simulink model "NPPF_N2_TH4"  (Simulink 10.0)
settings: Solver=VariableStepAuto  StartTime=0.0  StopTime=50  RelTol=1e-3
undefined symbols (not defined in the file): AL1, AL2, AT1, AT2, b, d, disturbance, g, Ix, Iy, Iz, l, m, P1, P2, t_end, t_start
libraries: truetime x3, simulink x3
settings Model: Creator=sunny  LastModifiedBy=peter
settings DataIOCC: LimitDataPoints=on  SignalLoggingSaveFormat=ModelDataLogs
settings OptimizationCC: BlockReduction=off  BooleanDataType=off
settings DebuggingCC: SaveWithParameterizedLinksMsg=none  SignalResolutionControl=TryResolveAllWithWarning  MultiTaskDSMMsg=warning  MultiTaskCondExecSysMsg=none  StateNameClashWarn=warning
settings HardwareCC: TargetBitPerPointer=64  TargetBitPerSizeT=64  TargetBitPerPtrDiffT=64  TargetLongLongMode=on  TargetIntDivRoundTo=Zero  TargetEndianess=LittleEndian  TargetWordSize=64  TargetHWDeviceType=MATLAB Host  ProdEqTarget=off
settings GRTTargetCC: CombineOutputUpdateFcns=on  GRTInterface=off
settings ConfigComp: CovExternalEMLEnable=off

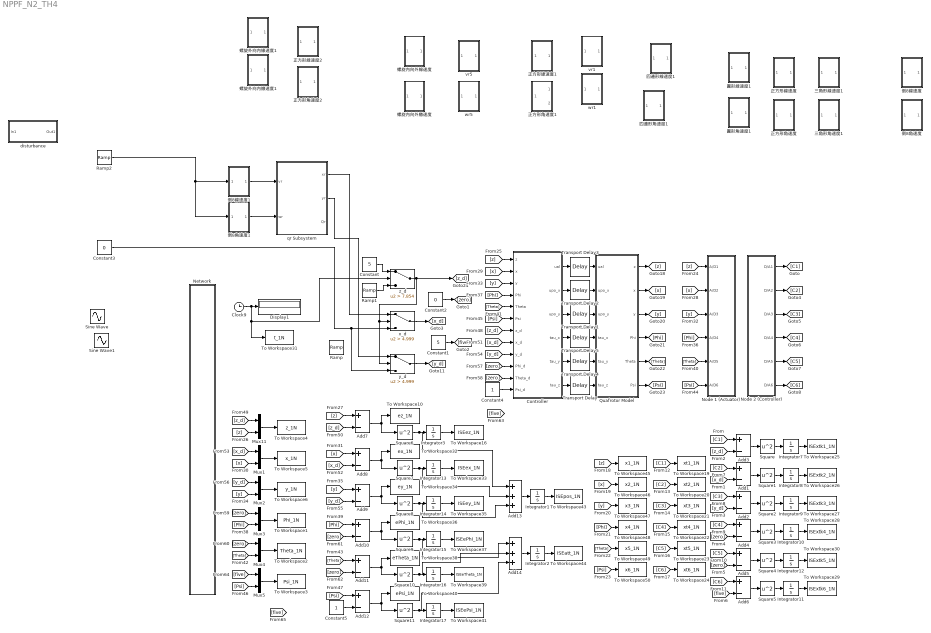
== system NPPF_N2_TH4 ==
  Add{1..12} (12 alike) : Sum  Inputs=+-
  Add13 : Sum  Inputs=+++
  Add14 : Sum  Inputs=+++
  Clock9 : Clock
  Constant : Constant  Value=5
  Constant1 : Constant  Value=5
  Constant2 : Constant  Value=0
  Constant3 : Constant  Value=0
  Constant4 : Constant
  Constant5 : Constant
  Controller : Subsystem
  Display1 : Display
  Integrator{1..3,7..17} (14 alike) : Integrator
  Mux{1..5,11} (6 alike) : Mux  Inputs=2
  Network : Subsystem
  Node 1 (Actuator) : Subsystem
  Node 2 (Controller) : Subsystem
  Quafrotor Model : Subsystem
  Ramp : simulink/Sources/Ramp  slope=0.5858/7.854  start=0  InitialOutput=0
  Ramp1 : simulink/Sources/Ramp  slope=5/7.854  start=0  InitialOutput=0
  Ramp2 : simulink/Sources/Ramp  slope=1  start=0  InitialOutput=0
  Sine Wave : Sin  Amplitude=2  Bias=2  Frequency=0.5  Phase=pi/2  SampleTime=0
  Sine Wave1 : Sin  Amplitude=2  Bias=2  Frequency=0.5  SampleTime=0
  Square{,1..11} (12 alike) : Math  Operator=square  SaturateOnIntegerOverflow=on
  To Workspace1 : ToWorkspace  VariableName=Phi_1N  SampleTime=-1
  To Workspace10 : ToWorkspace  VariableName=ez_1N  SampleTime=-1
  To Workspace16 : ToWorkspace  VariableName=ISEez_1N  SampleTime=-1
  To Workspace19 : ToWorkspace  VariableName=xt1_1N  SampleTime=-1
  To Workspace2 : ToWorkspace  VariableName=Theta_1N  SampleTime=-1
  To Workspace20 : ToWorkspace  VariableName=xt2_1N  SampleTime=-1
  To Workspace21 : ToWorkspace  VariableName=xt3_1N  SampleTime=-1
  To Workspace22 : ToWorkspace  VariableName=xt4_1N  SampleTime=-1
  To Workspace23 : ToWorkspace  VariableName=xt5_1N  SampleTime=-1
  To Workspace24 : ToWorkspace  VariableName=xt6_1N  SampleTime=-1
  To Workspace25 : ToWorkspace  VariableName=ISExtk1_1N  SampleTime=-1
  To Workspace26 : ToWorkspace  VariableName=ISExtk2_1N  SampleTime=-1
  To Workspace27 : ToWorkspace  VariableName=ISExtk3_1N  SampleTime=-1
  To Workspace28 : ToWorkspace  VariableName=ISExtk4_1N  SampleTime=-1
  To Workspace29 : ToWorkspace  VariableName=ISExtk6_1N  SampleTime=-1
  To Workspace3 : ToWorkspace  VariableName=Psi_1N  SampleTime=-1
  To Workspace30 : ToWorkspace  VariableName=ISExtk5_1N  SampleTime=-1
  To Workspace31 : ToWorkspace  VariableName=t_1N  SampleTime=-1
  To Workspace32 : ToWorkspace  VariableName=ex_1N  SampleTime=-1
  To Workspace33 : ToWorkspace  VariableName=ISEex_1N  SampleTime=-1
  To Workspace34 : ToWorkspace  VariableName=ey_1N  SampleTime=-1
  To Workspace35 : ToWorkspace  VariableName=ISEey_1N  SampleTime=-1
  To Workspace36 : ToWorkspace  VariableName=ePhi_1N  SampleTime=-1
  To Workspace37 : ToWorkspace  VariableName=ISEePhi_1N  SampleTime=-1
  To Workspace38 : ToWorkspace  VariableName=eTheta_1N  SampleTime=-1
  To Workspace39 : ToWorkspace  VariableName=ISEeTheta_1N  SampleTime=-1
  To Workspace4 : ToWorkspace  VariableName=z_1N  SampleTime=-1
  To Workspace40 : ToWorkspace  VariableName=ePsi_1N  SampleTime=-1
  To Workspace41 : ToWorkspace  VariableName=ISEePsi_1N  SampleTime=-1
  To Workspace43 : ToWorkspace  VariableName=ISEpos_1N  SampleTime=-1
  To Workspace44 : ToWorkspace  VariableName=ISEatt_1N  SampleTime=-1
  To Workspace45 : ToWorkspace  VariableName=x1_1N  SampleTime=-1
  To Workspace46 : ToWorkspace  VariableName=x2_1N  SampleTime=-1
  To Workspace47 : ToWorkspace  VariableName=x3_1N  SampleTime=-1
  To Workspace48 : ToWorkspace  VariableName=x4_1N  SampleTime=-1
  To Workspace49 : ToWorkspace  VariableName=x5_1N  SampleTime=-1
  To Workspace5 : ToWorkspace  VariableName=x_1N  SampleTime=-1
  To Workspace50 : ToWorkspace  VariableName=x6_1N  SampleTime=-1
  To Workspace6 : ToWorkspace  VariableName=y_1N  SampleTime=-1
  Transport Delay{,1..5} (6 alike) : TransportDelay
  disturbance : Subsystem
  qr Subsystem : Subsystem
  vr1 : Subsystem
  vr5 : Subsystem
  wr1 : Subsystem
  wr5 : Subsystem
  x_d : Switch  Criteria=u2 > Threshold  Threshold=4.999
  y_d : Switch  Criteria=u2 > Threshold  Threshold=4.999
  z_d : Switch  Criteria=u2 > Threshold  Threshold=7.854
  三角形線速度1 : Subsystem
  三角形角速度1 : Subsystem
  倒8線速度 : Subsystem
  倒8線速度1 : Subsystem
  倒8角速度 : Subsystem
  倒8角速度1 : Subsystem
  四邊形線速度1 : Subsystem
  四邊形角速度1 : Subsystem
  圓形線速度1 : Subsystem
  圓形角速度1 : Subsystem
  正方形線速度 : Subsystem
  正方形線速度1 : Subsystem
  正方形線速度2 : Subsystem
  正方形角速度 : Subsystem
  正方形角速度1 : Subsystem
  正方形角速度2 : Subsystem
  螺旋內向外線速度 : Subsystem
  螺旋內向外繳速度 : Subsystem
  螺旋外向內線速度1 : Subsystem
  螺旋外向內繳速度1 : Subsystem
  wires:
  Ramp1/1 -> z_d/3
  Constant/1 -> z_d/1
  Clock9/1 -> To Workspace31/1, z_d/2, Display1/1
  Controller/1(ual) -> Transport Delay3/1
  Controller/6(tau_z) -> Transport Delay/1
  Controller/5(tau_y) -> Transport Delay4/1
  Controller/4(tau_x) -> Transport Delay5/1
  Controller/3(upo_y) -> Transport Delay1/1
  Controller/2(upo_x) -> Transport Delay2/1
  Mux11/1 -> To Workspace4/1
  Integrator7/1 -> To Workspace25/1
  Square/1 -> Integrator7/1
  Add3/1 -> Square/1
  Add1/1 -> Square1/1
  Square1/1 -> Integrator8/1
  Integrator8/1 -> To Workspace26/1
  Square2/1 -> Integrator9/1
  Integrator9/1 -> To Workspace27/1
  Add2/1 -> Square2/1
  Integrator10/1 -> To Workspace28/1
  Square3/1 -> Integrator10/1
  Add4/1 -> Square3/1
  Add5/1 -> Square4/1
  Square4/1 -> Integrator12/1
  Integrator12/1 -> To Workspace30/1
  Add6/1 -> Square5/1
  Integrator11/1 -> To Workspace29/1
  Square5/1 -> Integrator11/1
  Integrator3/1 -> To Workspace16/1
  Square6/1 -> Add13/1, Integrator3/1
  Add7/1 -> Square6/1, To Workspace10/1
  Square7/1 -> Add13/2, Integrator13/1
  Add8/1 -> Square7/1, To Workspace32/1
  Integrator13/1 -> To Workspace33/1
  Integrator14/1 -> To Workspace35/1
  Square8/1 -> Add13/3, Integrator14/1
  Add9/1 -> Square8/1, To Workspace34/1
  Integrator15/1 -> To Workspace37/1
  Square9/1 -> Add14/1, Integrator15/1
  Add10/1 -> Square9/1, To Workspace36/1
  Integrator16/1 -> To Workspace39/1
  Square10/1 -> Add14/2, Integrator16/1
  Add11/1 -> Square10/1, To Workspace38/1
  Integrator17/1 -> To Workspace41/1
  Square11/1 -> Add14/3, Integrator17/1
  Add12/1 -> Square11/1, To Workspace40/1
  [z_d] -> Add3/2
  Node 2 (Controller)/1(D/A1) -> [C1]
  Node 2 (Controller)/2(D/A2) -> [C2]
  Node 2 (Controller)/3(D/A3) -> [C3]
  Node 2 (Controller)/4(D/A4) -> [C4]
  Node 2 (Controller)/5(D/A5) -> [C5]
  Node 2 (Controller)/6(D/A6) -> [C6]
  [C1] -> Add3/1
  [x_d] -> Add1/2
  [C2] -> Add1/1
  [C3] -> Add2/1
  [y_d] -> Add2/2
  [C4] -> Add4/1
  [zero] -> Add4/2
  [C5] -> Add5/1
  [zero] -> Add5/2
  [C6] -> Add6/1
  [five] -> Add6/2
  [C1] -> To Workspace19/1
  [C2] -> To Workspace20/1
  [C3] -> To Workspace21/1
  [C4] -> To Workspace22/1
  [C5] -> To Workspace23/1
  [C6] -> To Workspace24/1
  Quafrotor Model/1(z) -> [z]
  [z] -> Node 1 (Actuator)/1(A/D1)
  [z] -> Controller/1(z)
  [z] -> Mux11/2
  [z] -> Add7/1
  Quafrotor Model/2(x) -> [x]
  [x] -> Node 1 (Actuator)/2(A/D2)
  [x] -> Controller/2(x)
  [x] -> Add8/1
  Quafrotor Model/3(y) -> [y]
  [y] -> Node 1 (Actuator)/3(A/D3)
  [y] -> Controller/3(y)
  [y] -> Add9/1
  Quafrotor Model/4(Phi) -> [Phi]
  [Phi] -> Node 1 (Actuator)/4(A/D4)
  [Phi] -> Controller/4(Phi)
  [Phi] -> Add10/1
  Quafrotor Model/5(Theta) -> [Theta]
  [Theta] -> Node 1 (Actuator)/5(A/D5)
  [Theta] -> Controller/5(Theta)
  [Theta] -> Add11/1
  Quafrotor Model/6(Psi) -> [Psi]
  [Psi] -> Node 1 (Actuator)/6(A/D6)
  [Psi] -> Controller/6("Psi ")
  [Psi] -> Add12/1
  z_d/1 -> [z_d], y_d/2, x_d/2
  [z_d] -> Controller/7(z_d)
  [z_d] -> Mux11/1
  [z_d] -> Add7/2
  x_d/1 -> [x_d]
  [x_d] -> Controller/8(x_d)
  [x_d] -> Add8/2
  y_d/1 -> [y_d]
  [y_d] -> Controller/9(y_d)
  [y_d] -> Add9/2
  Constant2/1 -> [zero]
  Constant1/1 -> [five]
  [zero] -> Controller/10(Phi_d)
  [zero] -> Controller/11(Theta_d)
  [zero] -> Add10/2
  [zero] -> Add11/2
  Constant4/1 -> Controller/12(Psi_d)
  Constant5/1 -> Add12/2
  [x_d] -> Mux1/1
  Mux1/1 -> To Workspace5/1
  [x] -> Mux1/2
  [y_d] -> Mux2/1
  Mux2/1 -> To Workspace6/1
  [y] -> Mux2/2
  [zero] -> Mux3/1
  Mux3/1 -> To Workspace1/1
  [Phi] -> Mux3/2
  [zero] -> Mux4/1
  Mux4/1 -> To Workspace2/1
  [Theta] -> Mux4/2
  [five] -> Mux5/1
  Mux5/1 -> To Workspace3/1
  [Psi] -> Mux5/2
  Add13/1 -> Integrator1/1
  Integrator1/1 -> To Workspace43/1
  Add14/1 -> Integrator2/1
  Integrator2/1 -> To Workspace44/1
  [Psi] -> To Workspace50/1
  [z] -> To Workspace45/1
  [Phi] -> To Workspace48/1
  [y] -> To Workspace47/1
  [Theta] -> To Workspace49/1
  [x] -> To Workspace46/1
  倒8線速度1/1(Out1) -> qr Subsystem/1(vr)
  倒8角速度1/1(Out1) -> qr Subsystem/2(wr)
  Constant3/1 -> y_d/3, x_d/3
  qr Subsystem/1(xr) -> x_d/1
  qr Subsystem/2(yr) -> y_d/1
  Ramp2/1 -> 倒8角速度1/1(In2), 倒8線速度1/1(In2)
  Transport Delay3/1 -> Quafrotor Model/1(ual)
  Transport Delay2/1 -> Quafrotor Model/2(upo_x)
  Transport Delay1/1 -> Quafrotor Model/3(upo_y)
  Transport Delay5/1 -> Quafrotor Model/4(tau_x)
  Transport Delay4/1 -> Quafrotor Model/5(tau_y)
  Transport Delay/1 -> Quafrotor Model/6(tau_z)

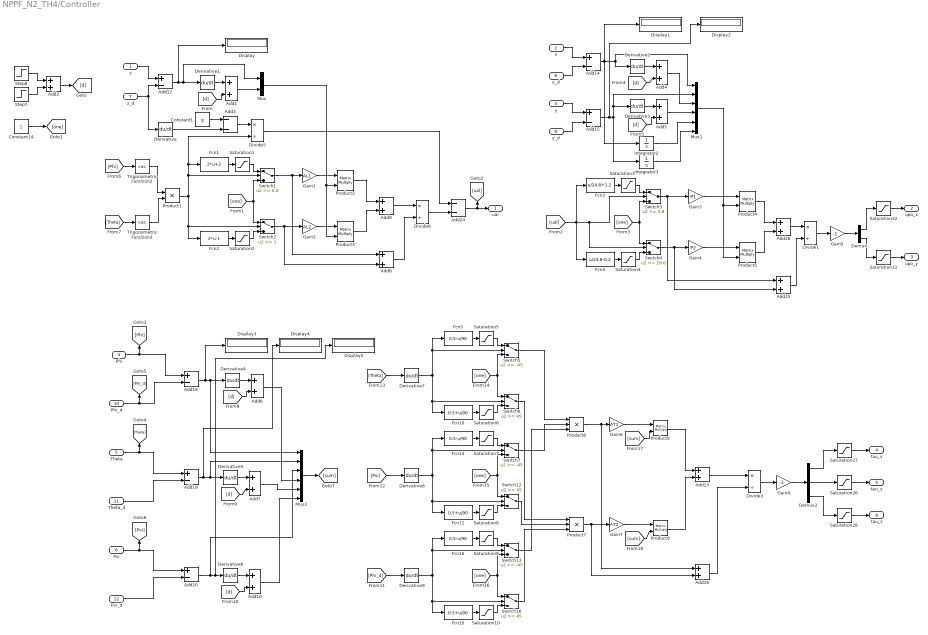
== system NPPF_N2_TH4/Controller ==
  z : Inport
  x : Inport  Port=2
  y : Inport  Port=3
  Phi : Inport  Port=4
  Theta : Inport  Port=5
  "Psi " : Inport  Port=6
  z_d : Inport  Port=7
  x_d : Inport  Port=8
  y_d : Inport  Port=9
  Phi_d : Inport  Port=10
  Theta_d : Inport  Port=11
  Psi_d : Inport  Port=12
  Add{1..2,4..10,13,16,25..26} (13 alike) : Sum
  Add{12,14..15,18..20} (6 alike) : Sum  Inputs=+-
  Add24 : Sum  Inputs=--
  Add3 : Sum  Inputs=--
  Constant1 : Constant  Value=g
  Constant14 : Constant
  Demux : Demux  Outputs=2
  Demux2 : Demux  Outputs=3
  Derivative{,1..9} (10 alike) : Derivative
  Display{,1..5} (6 alike) : Display
  Divide{1,3,5..6} (4 alike) : Product  Inputs=*/
  Fcn1 : Fcn  Expr=2*u+2
  Fcn10 : Fcn  Expr=0.5+u/90
  Fcn11 : Fcn  Expr=0.5+u/90
  Fcn14 : Fcn  Expr=0.5-u/90
  Fcn15 : Fcn  Expr=0.5+u/90
  Fcn16 : Fcn  Expr=0.5-u/90
  Fcn2 : Fcn  Expr=2*u-1
  Fcn3 : Fcn  Expr=u/24.8+1.2
  Fcn4 : Fcn  Expr=u/24.8-0.2
  Fcn5 : Fcn  Expr=0.5-u/90
  Gain1 : Gain  Gain=AL1
  Gain2 : Gain  Gain=AL2
  Gain3 : Gain  Gain=P1
  Gain4 : Gain  Gain=P2
  Gain5 : Gain  Gain=-1
  Gain6 : Gain  Gain=AT1
  Gain7 : Gain  Gain=AT2
  Gain8 : Gain  Gain=-1
  Integrator2 : Integrator
  Integrator3 : Integrator
  Mux : Mux  Inputs=2
  Mux1 : Mux  Inputs=6
  Mux2 : Mux  Inputs=6
  Product1 : Product
  Product{2..5,8..9} (6 alike) : Product  Multiplication=Matrix(*)  RndMeth=Zero
  Product6 : Product  Inputs=3
  Product7 : Product  Inputs=3
  Saturation{1..10} (10 alike) : Saturate  UpperLimit=1  LowerLimit=0
  Saturation{26..28,31..32} (5 alike) : Saturate  UpperLimit=2000  LowerLimit=-2000
  Step7 : Step  Time=t_start  After=disturbance  SampleTime=0
  Step8 : Step  Time=t_end  After=-disturbance  SampleTime=0
  Switch1 : Switch  Threshold=0.5
  Switch12 : Switch  Threshold=45
  Switch13 : Switch  Threshold=-45
  Switch16 : Switch  Threshold=45
  Switch2 : Switch  Threshold=1
  Switch3 : Switch  Threshold=4.8
  Switch4 : Switch  Threshold=29.6
  Switch5 : Switch  Threshold=-45
  Switch6 : Switch  Threshold=45
  Switch7 : Switch  Threshold=-45
  Trigonometric Function2 : Trigonometry  Operator=cos
  Trigonometric Function3 : Trigonometry  Operator=cos
  ual : Outport  VectorParamsAs1DForOutWhenUnconnected=off
  upo_x : Outport  Port=2  VectorParamsAs1DForOutWhenUnconnected=off
  upo_y : Outport  Port=3  VectorParamsAs1DForOutWhenUnconnected=off
  tau_x : Outport  Port=4  VectorParamsAs1DForOutWhenUnconnected=off
  tau_y : Outport  Port=5  VectorParamsAs1DForOutWhenUnconnected=off
  tau_z : Outport  Port=6  VectorParamsAs1DForOutWhenUnconnected=off
  wires:
  Saturation32/1 -> upo_x/1
  Saturation31/1 -> upo_y/1
  z/1 -> Add12/1
  z_d/1 -> Derivative/1, Add12/2
  Add12/1 -> Display/1, Mux/1, Derivative1/1
  Add2/1 -> [d]
  Trigonometric Function2/1 -> Product1/1
  Trigonometric Function3/1 -> Product1/2
  Derivative/1 -> Add3/2
  Constant1/1 -> Add3/1
  Add3/1 -> Divide5/1
  Fcn1/1 -> Saturation1/1
  Saturation1/1 -> Switch1/1
  [one] -> Switch1/3, Switch2/1
  Fcn2/1 -> Saturation2/1
  Saturation2/1 -> Switch2/3
  Product1/1 -> Switch1/2, Fcn1/1, Divide5/2, Fcn2/1, Switch2/2
  Constant14/1 -> [one]
  Switch1/1 -> Add8/1, Gain1/1
  Switch2/1 -> Add8/2, Gain2/1
  Gain1/1 -> Product2/1
  Gain2/1 -> Product3/1
  Mux/1 -> Product3/2, Product2/2
  Product2/1 -> Add9/1
  Product3/1 -> Add9/2
  Add9/1 -> Divide6/1
  Add8/1 -> Divide6/2
  Divide5/1 -> Add24/1
  Divide6/1 -> Add24/2
  Add24/1 -> [ual], ual/1
  Fcn4/1 -> Saturation4/1
  [one] -> Switch3/3, Switch4/1
  Saturation3/1 -> Switch3/1
  Fcn3/1 -> Saturation3/1
  [ual] -> Switch4/2, Switch3/2, Fcn4/1, Fcn3/1
  Saturation4/1 -> Switch4/3
  x/1 -> Add14/1
  x_d/1 -> Add14/2
  y/1 -> Add15/1
  y_d/1 -> Add15/2
  Integrator2/1 -> Mux1/5
  Integrator3/1 -> Mux1/6
  Switch3/1 -> Gain3/1, Add25/1
  Switch4/1 -> Add25/2, Gain4/1
  Gain3/1 -> Product4/1
  Gain4/1 -> Product5/1
  Mux1/1 -> Product4/2, Product5/2
  Product5/1 -> Add26/2
  Divide1/1 -> Gain5/1
  Product4/1 -> Add26/1
  Add26/1 -> Divide1/1
  Add25/1 -> Divide1/2
  Gain5/1 -> Demux/1
  Demux/1 -> Saturation32/1
  Demux/2 -> Saturation31/1
  [Phi] -> Trigonometric Function2/1
  [Theta] -> Trigonometric Function3/1
  Phi/1 -> Add18/1, [Phi]
  Theta/1 -> Add19/1, [Theta]
  Phi_d/1 -> [Phi_d], Add18/2
  Theta_d/1 -> Add19/2
  "Psi "/1 -> [Psi], Add20/1
  Psi_d/1 -> Add20/2
  [Theta] -> Derivative7/1
  [Psi] -> Derivative8/1
  [Phi_d] -> Derivative9/1
  Derivative7/1 -> Switch5/2, Fcn5/1, Fcn10/1, Switch6/2
  Fcn10/1 -> Saturation6/1
  Saturation5/1 -> Switch5/1
  Fcn5/1 -> Saturation5/1
  Saturation6/1 -> Switch6/3
  [one] -> Switch5/3, Switch6/1
  Saturation8/1 -> Switch12/3
  [one] -> Switch7/3, Switch12/1
  Saturation7/1 -> Switch7/1
  Fcn11/1 -> Saturation8/1
  Derivative8/1 -> Switch7/2, Fcn14/1, Fcn11/1, Switch12/2
  Fcn14/1 -> Saturation7/1
  Saturation10/1 -> Switch16/3
  [one] -> Switch13/3, Switch16/1
  Saturation9/1 -> Switch13/1
  Fcn15/1 -> Saturation10/1
  Derivative9/1 -> Switch13/2, Fcn16/1, Fcn15/1, Switch16/2
  Fcn16/1 -> Saturation9/1
  Product6/1 -> Add16/1, Gain6/1
  Product7/1 -> Add16/2, Gain7/1
  Switch5/1 -> Product6/1
  Switch7/1 -> Product6/2
  Switch13/1 -> Product6/3
  Switch6/1 -> Product7/1
  Switch12/1 -> Product7/2
  Switch16/1 -> Product7/3
  Gain6/1 -> Product8/1
  Gain7/1 -> Product9/1
  Product8/1 -> Add13/1
  Product9/1 -> Add13/2
  Add13/1 -> Divide3/1
  Add16/1 -> Divide3/2
  Divide3/1 -> Gain8/1
  Gain8/1 -> Demux2/1
  Demux2/2 -> Saturation26/1
  Demux2/1 -> Saturation27/1
  Demux2/3 -> Saturation28/1
  Saturation27/1 -> tau_x/1
  Saturation26/1 -> tau_y/1
  Saturation28/1 -> tau_z/1
  [sum] -> Product8/2
  [sum] -> Product9/2
  Mux2/1 -> [sum]
  [d] -> Add1/2
  Derivative1/1 -> Add1/1
  Add1/1 -> Mux/2
  [d] -> Add4/2
  Derivative2/1 -> Add4/1
  Add14/1 -> Display1/1, Mux1/1, Derivative2/1, Integrator2/1
  Add4/1 -> Mux1/3
  [d] -> Add5/2
  Derivative3/1 -> Add5/1
  Add15/1 -> Display2/1, Mux1/2, Derivative3/1, Integrator3/1
  Add5/1 -> Mux1/4
  [d] -> Add6/2
  Derivative4/1 -> Add6/1
  Add18/1 -> Display3/1, Mux2/1, Derivative4/1
  Add6/1 -> Mux2/4
  [d] -> Add7/2
  Derivative5/1 -> Add7/1
  Add19/1 -> Display4/1, Mux2/2, Derivative5/1
  Add7/1 -> Mux2/5
  [d] -> Add10/2
  Derivative6/1 -> Add10/1
  Add20/1 -> Display5/1, Derivative6/1, Mux2/3
  Add10/1 -> Mux2/6
  Step7/1 -> Add2/2
  Step8/1 -> Add2/1

== system NPPF_N2_TH4/Network ==
  Terminator : Terminator
  TrueTime Network : truetime/TrueTime Network  nwtype=CSMA/CD (Ethernet)  nwnbr=1  nnodes=2  rate=10000000  minsize=512  lossprob=0.6  seed=0  bandwidths=[0.5 0.5]  slotsize=512  schedule=[1 1 2]  memsize=80000  buftype=Common buffer  overflow=Retransmit  dynSchedule=0  miniSlotSize=0  NIT=0  QSortMode=FIFO  sync=0  irtSchedule=0  nrtLength=0  nodeGraph=0  scheduleoutput=on
  wires:
  TrueTime Network/1 -> Terminator/1

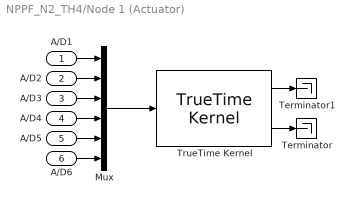
== system NPPF_N2_TH4/Node 1 (Actuator) ==
  A/D1 : Inport
  A/D2 : Inport  Port=2
  A/D3 : Inport  Port=3
  A/D4 : Inport  Port=4
  A/D5 : Inport  Port=5
  A/D6 : Inport  Port=6
  Mux : Mux  Inputs=6
  Terminator : Terminator
  Terminator1 : Terminator
  TrueTime Kernel : truetime/TrueTime Kernel  sfun=actuator_init  args=[]  ninputsoutputs=[6 6]  ntriggers=0  trigtype=falling  nwnodenbr=1  clockoffsetdrift=[0 0]  schedoutput=on  battery=off  poweroutput=off  label=1: 1
  wires:
  TrueTime Kernel/1 -> Terminator1/1
  A/D1/1 -> Mux/1
  A/D2/1 -> Mux/2
  A/D3/1 -> Mux/3
  Mux/1 -> TrueTime Kernel/1
  A/D4/1 -> Mux/4
  A/D5/1 -> Mux/5
  A/D6/1 -> Mux/6
  TrueTime Kernel/2 -> Terminator/1

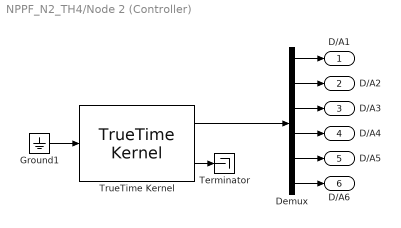
== system NPPF_N2_TH4/Node 2 (Controller) ==
  Demux : Demux  Outputs=6
  Ground1 : Ground
  Terminator : Terminator
  TrueTime Kernel : truetime/TrueTime Kernel  sfun=controllertest_init  args=[]  ninputsoutputs=[1 6]  ntriggers=0  trigtype=falling  nwnodenbr=2  clockoffsetdrift=[0 0]  schedoutput=on  battery=off  poweroutput=off  label=1: 2
  D/A1 : Outport  VectorParamsAs1DForOutWhenUnconnected=off
  D/A2 : Outport  Port=2  VectorParamsAs1DForOutWhenUnconnected=off
  D/A3 : Outport  Port=3  VectorParamsAs1DForOutWhenUnconnected=off
  D/A4 : Outport  Port=4  VectorParamsAs1DForOutWhenUnconnected=off
  D/A5 : Outport  Port=5  VectorParamsAs1DForOutWhenUnconnected=off
  D/A6 : Outport  Port=6  VectorParamsAs1DForOutWhenUnconnected=off
  wires:
  TrueTime Kernel/1 -> Demux/1
  Ground1/1 -> TrueTime Kernel/1
  Demux/1 -> D/A1/1
  Demux/2 -> D/A2/1
  Demux/3 -> D/A3/1
  Demux/4 -> D/A4/1
  Demux/5 -> D/A5/1
  Demux/6 -> D/A6/1
  TrueTime Kernel/2 -> Terminator/1

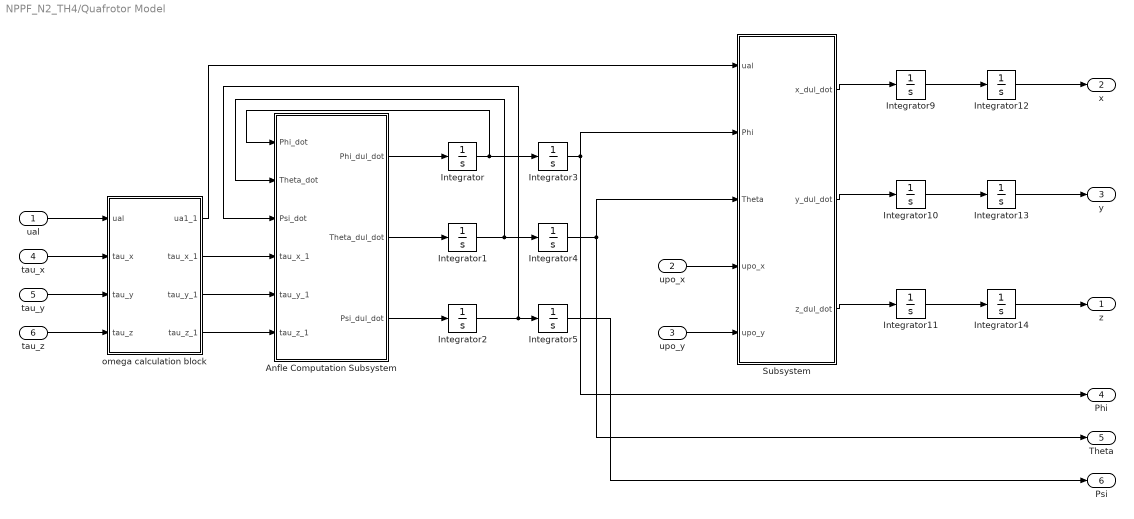
== system NPPF_N2_TH4/Quafrotor Model ==
  ual : Inport
  upo_x : Inport  Port=2
  upo_y : Inport  Port=3
  tau_x : Inport  Port=4
  tau_y : Inport  Port=5
  tau_z : Inport  Port=6
  Anfle Computation Subsystem : Subsystem
  Integrator{,1..5,9..14} (12 alike) : Integrator
  Subsystem : Subsystem
  omega calculation block : Subsystem
  z : Outport  VectorParamsAs1DForOutWhenUnconnected=off
  x : Outport  Port=2  VectorParamsAs1DForOutWhenUnconnected=off
  y : Outport  Port=3  VectorParamsAs1DForOutWhenUnconnected=off
  Phi : Outport  Port=4  VectorParamsAs1DForOutWhenUnconnected=off
  Theta : Outport  Port=5  VectorParamsAs1DForOutWhenUnconnected=off
  Psi : Outport  Port=6  VectorParamsAs1DForOutWhenUnconnected=off
  wires:
  tau_y/1 -> omega calculation block/3(tau_y)
  Integrator2/1 -> Anfle Computation Subsystem/3(Psi_dot), Integrator5/1
  Integrator3/1 -> Phi/1, Subsystem/2(Phi)
  Integrator11/1 -> Integrator14/1
  tau_x/1 -> omega calculation block/2(tau_x)
  tau_z/1 -> omega calculation block/4(tau_z)
  Integrator5/1 -> Psi/1
  Integrator1/1 -> Integrator4/1, Anfle Computation Subsystem/2(Theta_dot)
  Integrator4/1 -> Theta/1, Subsystem/3(Theta)
  Integrator14/1 -> z/1
  omega calculation block/1(ua1_1) -> Subsystem/1(ual)
  Integrator9/1 -> Integrator12/1
  Integrator10/1 -> Integrator13/1
  Subsystem/1(x_dul_dot) -> Integrator9/1
  Subsystem/3(z_dul_dot) -> Integrator11/1
  omega calculation block/2(tau_x_1) -> Anfle Computation Subsystem/4(tau_x_1)
  Anfle Computation Subsystem/3(Psi_dul_dot) -> Integrator2/1
  Anfle Computation Subsystem/2(Theta_dul_dot) -> Integrator1/1
  omega calculation block/4(tau_z_1) -> Anfle Computation Subsystem/6(tau_z_1)
  Integrator/1 -> Anfle Computation Subsystem/1(Phi_dot), Integrator3/1
  ual/1 -> omega calculation block/1(ual)
  omega calculation block/3(tau_y_1) -> Anfle Computation Subsystem/5(tau_y_1)
  Anfle Computation Subsystem/1(Phi_dul_dot) -> Integrator/1
  Integrator13/1 -> y/1
  Integrator12/1 -> x/1
  Subsystem/2(y_dul_dot) -> Integrator10/1
  upo_y/1 -> Subsystem/5(upo_y)
  upo_x/1 -> Subsystem/4(upo_x)

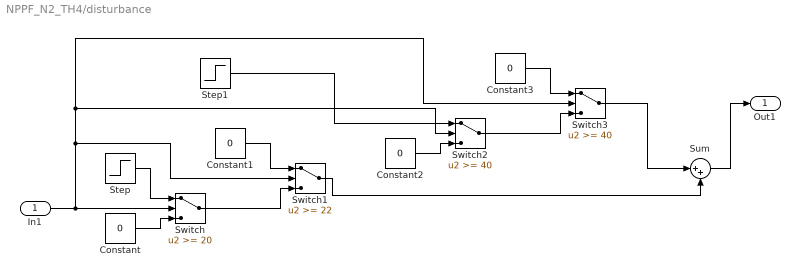
== system NPPF_N2_TH4/disturbance ==
  In1 : Inport
  Constant{,1..3} (4 alike) : Constant  Value=0
  Step : Step  After=-0.8  SampleTime=0
  Step1 : Step  After=0.4  SampleTime=0
  Sum : Sum  Inputs=|++
  Switch : Switch  Threshold=20  ZeroCross=off
  Switch1 : Switch  Threshold=22
  Switch2 : Switch  Threshold=40  ZeroCross=off
  Switch3 : Switch  Threshold=40
  Out1 : Outport
  wires:
  Constant/1 -> Switch/3
  Switch/1 -> Switch1/3
  Constant1/1 -> Switch1/1
  Step/1 -> Switch/1
  In1/1 -> Switch3/2, Switch2/2, Switch1/2, Switch/2
  Constant2/1 -> Switch2/3
  Switch2/1 -> Switch3/3
  Constant3/1 -> Switch3/1
  Switch1/1 -> Sum/2
  Switch3/1 -> Sum/1
  Sum/1 -> Out1/1
  Step1/1 -> Switch2/1

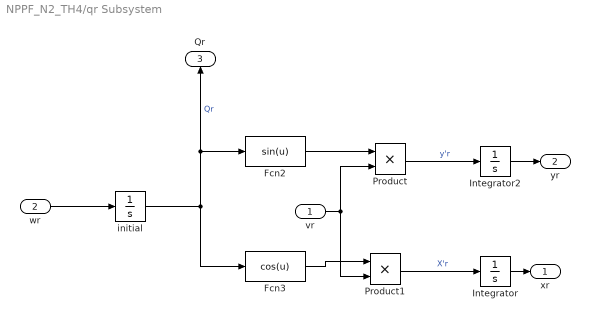
== system NPPF_N2_TH4/qr Subsystem ==
  vr : Inport
  wr : Inport  Port=2
  Fcn2 : Fcn  Expr=sin(u)
  Fcn3 : Fcn  Expr=cos(u)
  Integrator : Integrator
  Integrator2 : Integrator
  Product : Product  RndMeth=Zero
  Product1 : Product  RndMeth=Zero
  initial : Integrator  InitialCondition=0*pi/180
  xr : Outport
  yr : Outport  Port=2
  Qr : Outport  Port=3
  wires:
  Fcn2/1 -> Product/1
  initial/1 -> Fcn3/1, Qr/1, Fcn2/1  "Qr"
  Product1/1 -> Integrator/1  "X'r"
  wr/1 -> initial/1
  Integrator2/1 -> yr/1
  Integrator/1 -> xr/1
  vr/1 -> Product/2, Product1/2
  Product/1 -> Integrator2/1  "y'r"
  Fcn3/1 -> Product1/1

== system NPPF_N2_TH4/vr1 ==
  In1 : Inport
  02V : DiscretePulseGenerator  PulseType=Time based  Amplitude=0.1  Period=12  PulseWidth=300/12  PhaseDelay=7
  04V : DiscretePulseGenerator  PulseType=Time based  Amplitude=0.4  Period=12  PulseWidth=900/12
  Add : Sum
  Fcn1 : Fcn  Expr=0.4
  Scope : Scope
  Out1 : Outport
  wires:
  In1/1 -> Fcn1/1
  04V/1 -> Add/1
  02V/1 -> Add/2
  Add/1 -> Scope/1, Out1/1

== system NPPF_N2_TH4/vr5 ==
  In1 : Inport
  02V : DiscretePulseGenerator  PulseType=Time based  Amplitude=0  Period=12  PulseWidth=300/12
  04V : DiscretePulseGenerator  PulseType=Time based  Amplitude=0.4  Period=12  PulseWidth=900/12
  Add : Sum
  Fcn1 : Fcn  Expr=0.4
  Scope : Scope
  Out1 : Outport
  wires:
  In1/1 -> Fcn1/1
  04V/1 -> Add/1
  02V/1 -> Add/2
  Add/1 -> Scope/1, Out1/1

== system NPPF_N2_TH4/wr1 ==
  In1 : Inport
  02V : DiscretePulseGenerator  PulseType=Time based  Amplitude=0.2  PulseWidth=50  PhaseDelay=1
  04V : DiscretePulseGenerator  PulseType=Time based  Amplitude=90*3.14159/180  Period=12  PulseWidth=300/12  PhaseDelay=7
  Fcn1 : Fcn  Expr=3*sin(0.05*u)
  Scope : Scope
  Out1 : Outport
  wires:
  In1/1 -> Fcn1/1
  04V/1 -> Scope/1, Out1/1

== system NPPF_N2_TH4/wr5 ==
  In1 : Inport
  02V : DiscretePulseGenerator  PulseType=Time based  Amplitude=0.2  PulseWidth=50  PhaseDelay=1
  04V : DiscretePulseGenerator  PulseType=Time based  Amplitude=90*pi/180  Period=12  PulseWidth=300/12  PhaseDelay=9
  Fcn1 : Fcn  Expr=3*sin(0.05*u)
  Scope : Scope
  Out1 : Outport
  wires:
  In1/1 -> Fcn1/1
  04V/1 -> Scope/1, Out1/1

== system NPPF_N2_TH4/三角形線速度1 ==
  In1 : Inport
  02V : DiscretePulseGenerator  PulseType=Time based  Amplitude=0  Period=12  PulseWidth=400/12
  04V : DiscretePulseGenerator  PulseType=Time based  Amplitude=0.4  Period=12  PulseWidth=800/12
  Add : Sum
  Scope : Scope
  Out1 : Outport
  wires:
  04V/1 -> Add/1
  02V/1 -> Add/2
  Add/1 -> Scope/1, Out1/1

== system NPPF_N2_TH4/三角形角速度1 ==
  In1 : Inport
  04V : DiscretePulseGenerator  PulseType=Time based  Amplitude=120*pi/180  Period=12  PulseWidth=400/12  PhaseDelay=8
  Scope : Scope
  Out1 : Outport
  wires:
  04V/1 -> Scope/1, Out1/1

== system NPPF_N2_TH4/倒8線速度 ==
  In1 : Inport
  Fcn1 : Fcn  Expr=0.5
  Out1 : Outport
  wires:
  Fcn1/1 -> Out1/1
  In1/1 -> Fcn1/1

== system NPPF_N2_TH4/倒8線速度1 ==
  In2 : Inport
  Constant1 : Constant  Value=0.5
  Constant5 : Constant  Value=0
  Switch2 : Switch  Threshold=8  ZeroCross=off
  Out1 : Outport
  wires:
  Constant5/1 -> Switch2/3
  In2/1 -> Switch2/2
  Switch2/1 -> Out1/1
  Constant1/1 -> Switch2/1

== system NPPF_N2_TH4/倒8角速度 ==
  In1 : Inport
  Fcn1 : Fcn  Expr=-sin(2*pi*u/15.118)
  Out1 : Outport
  wires:
  Fcn1/1 -> Out1/1
  In1/1 -> Fcn1/1

== system NPPF_N2_TH4/倒8角速度1 ==
  In2 : Inport
  Constant5 : Constant  Value=0
  Fcn1 : Fcn  Expr=-sin(2*pi*u/15.118)
  Switch2 : Switch  Threshold=8  ZeroCross=off
  Out1 : Outport
  wires:
  Fcn1/1 -> Out1/1
  Switch2/1 -> Fcn1/1
  Constant5/1 -> Switch2/3
  In2/1 -> Switch2/1, Switch2/2

== system NPPF_N2_TH4/四邊形線速度1 ==
  In1 : Inport
  02V : DiscretePulseGenerator  PulseType=Time based  Amplitude=0.1  Period=11  PulseWidth=300/11  PhaseDelay=7
  04V : DiscretePulseGenerator  PulseType=Time based  Amplitude=0.4  Period=11  PulseWidth=700/11
  Add : Sum
  Fcn1 : Fcn  Expr=0.4
  Scope : Scope
  Out1 : Outport
  wires:
  In1/1 -> Fcn1/1
  04V/1 -> Add/1
  02V/1 -> Add/2
  Add/1 -> Scope/1, Out1/1

== system NPPF_N2_TH4/四邊形角速度1 ==
  In1 : Inport
  02V : DiscretePulseGenerator  PulseType=Time based  Amplitude=0.2  PulseWidth=50  PhaseDelay=1
  04V : DiscretePulseGenerator  PulseType=Time based  Amplitude=-30*3.14159/180  Period=11  PulseWidth=300/11  PhaseDelay=7
  Fcn1 : Fcn  Expr=3*sin(0.05*u)
  Scope : Scope
  Out1 : Outport
  wires:
  In1/1 -> Fcn1/1
  04V/1 -> Scope/1, Out1/1

== system NPPF_N2_TH4/圓形線速度1 ==
  In1 : Inport
  Fcn1 : Fcn  Expr=0.5
  Out1 : Outport
  wires:
  Fcn1/1 -> Out1/1
  In1/1 -> Fcn1/1

== system NPPF_N2_TH4/圓形角速度1 ==
  In1 : Inport
  Fcn1 : Fcn  Expr=0.5
  Out1 : Outport
  wires:
  Fcn1/1 -> Out1/1
  In1/1 -> Fcn1/1

== system NPPF_N2_TH4/正方形線速度 ==
  In1 : Inport
  02V : DiscretePulseGenerator  PulseType=Time based  Amplitude=0  Period=4  PulseWidth=25
  04V : DiscretePulseGenerator  PulseType=Time based  Amplitude=0.4  Period=4  PulseWidth=75
  Add : Sum
  Fcn1 : Fcn  Expr=0.4
  Scope : Scope
  Out1 : Outport
  wires:
  In1/1 -> Fcn1/1
  04V/1 -> Add/1
  02V/1 -> Add/2
  Add/1 -> Scope/1, Out1/1

== system NPPF_N2_TH4/正方形線速度1 ==
  In1 : Inport
  02V : DiscretePulseGenerator  PulseType=Time based  Amplitude=0  Period=12  PulseWidth=300/12
  04V : DiscretePulseGenerator  PulseType=Time based  Amplitude=0.4  Period=12  PulseWidth=900/12
  Add : Sum
  Fcn1 : Fcn  Expr=0.4
  Scope : Scope
  Out1 : Outport
  wires:
  In1/1 -> Fcn1/1
  04V/1 -> Add/1
  02V/1 -> Add/2
  Add/1 -> Scope/1, Out1/1

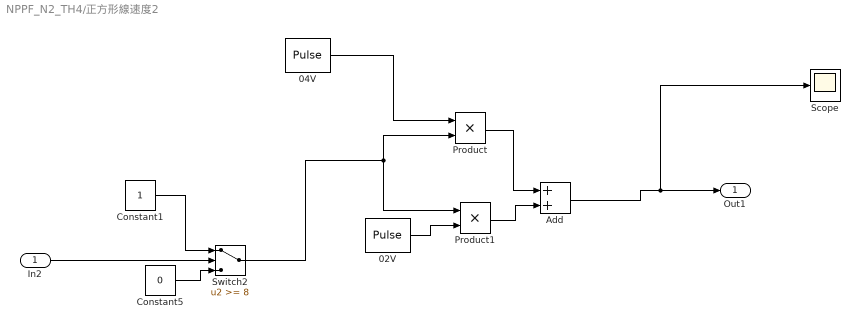
== system NPPF_N2_TH4/正方形線速度2 ==
  In2 : Inport
  02V : DiscretePulseGenerator  PulseType=Time based  Amplitude=0  Period=4  PulseWidth=25
  04V : DiscretePulseGenerator  PulseType=Time based  Amplitude=1.33  Period=4  PulseWidth=75
  Add : Sum
  Constant1 : Constant
  Constant5 : Constant  Value=0
  Product : Product
  Product1 : Product
  Scope : Scope
  Switch2 : Switch  Threshold=8  ZeroCross=off
  Out1 : Outport
  wires:
  Add/1 -> Scope/1, Out1/1
  04V/1 -> Product/1
  Switch2/1 -> Product1/1, Product/2
  Product/1 -> Add/1
  Product1/1 -> Add/2
  Constant1/1 -> Switch2/1
  Constant5/1 -> Switch2/3
  In2/1 -> Switch2/2
  02V/1 -> Product1/2

== system NPPF_N2_TH4/正方形角速度 ==
  In1 : Inport
  04V : DiscretePulseGenerator  PulseType=Time based  Amplitude=90*pi/180  Period=4  PulseWidth=25  PhaseDelay=3
  Scope : Scope
  Out1 : Outport
  wires:
  04V/1 -> Scope/1, Out1/1

== system NPPF_N2_TH4/正方形角速度1 ==
  In1 : Inport
  02V : DiscretePulseGenerator  PulseType=Time based  Amplitude=0.2  PulseWidth=50  PhaseDelay=1
  04V : DiscretePulseGenerator  PulseType=Time based  Amplitude=90*pi/180  Period=12  PulseWidth=300/12  PhaseDelay=9
  Fcn1 : Fcn  Expr=3*sin(0.05*u)
  Scope : Scope
  Out1 : Outport
  Out2 : Outport  Port=2
  wires:
  In1/1 -> Fcn1/1
  04V/1 -> Scope/1, Out1/1

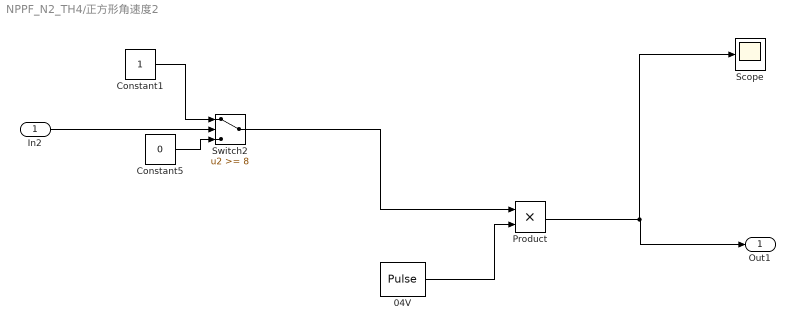
== system NPPF_N2_TH4/正方形角速度2 ==
  In2 : Inport
  04V : DiscretePulseGenerator  PulseType=Time based  Amplitude=90*pi/180  Period=4  PulseWidth=25  PhaseDelay=3
  Constant1 : Constant
  Constant5 : Constant  Value=0
  Product : Product
  Scope : Scope
  Switch2 : Switch  Threshold=8  ZeroCross=off
  Out1 : Outport
  wires:
  Switch2/1 -> Product/1
  04V/1 -> Product/2
  Product/1 -> Scope/1, Out1/1
  Constant5/1 -> Switch2/3
  Constant1/1 -> Switch2/1
  In2/1 -> Switch2/2

== system NPPF_N2_TH4/螺旋內向外線速度 ==
  In1 : Inport
  Fcn1 : Fcn  Expr=0.5
  Out1 : Outport
  wires:
  Fcn1/1 -> Out1/1
  In1/1 -> Fcn1/1

== system NPPF_N2_TH4/螺旋內向外繳速度 ==
  In1 : Inport
  Fcn1 : Fcn  Expr=1/(0.05*(u+10))
  Out1 : Outport
  wires:
  Fcn1/1 -> Out1/1
  In1/1 -> Fcn1/1

== system NPPF_N2_TH4/螺旋外向內線速度1 ==
  In1 : Inport
  Fcn1 : Fcn  Expr=0.5
  Out1 : Outport
  wires:
  Fcn1/1 -> Out1/1
  In1/1 -> Fcn1/1

== system NPPF_N2_TH4/螺旋外向內繳速度1 ==
  In1 : Inport
  Fcn1 : Fcn  Expr=0.015*u
  Out1 : Outport
  wires:
  Fcn1/1 -> Out1/1
  In1/1 -> Fcn1/1

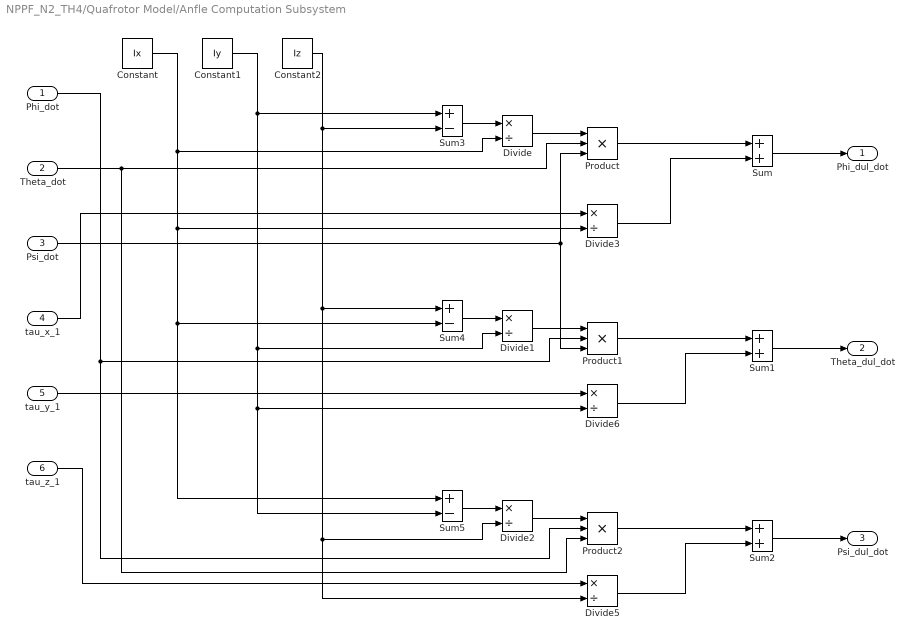
== system NPPF_N2_TH4/Quafrotor Model/Anfle Computation Subsystem ==
  Phi_dot : Inport
  Theta_dot : Inport  Port=2
  Psi_dot : Inport  Port=3
  tau_x_1 : Inport  Port=4
  tau_y_1 : Inport  Port=5
  tau_z_1 : Inport  Port=6
  Constant : Constant  Value=Ix
  Constant1 : Constant  Value=Iy
  Constant2 : Constant  Value=Iz
  Divide{,1..3,5..6} (6 alike) : Product  Inputs=*/
  Product : Product  Inputs=3
  Product1 : Product  Inputs=3
  Product2 : Product  Inputs=3
  Sum : Sum
  Sum1 : Sum
  Sum2 : Sum
  Sum3 : Sum  Inputs=+-
  Sum4 : Sum  Inputs=+-
  Sum5 : Sum  Inputs=+-
  Phi_dul_dot : Outport  VectorParamsAs1DForOutWhenUnconnected=off
  Theta_dul_dot : Outport  Port=2  VectorParamsAs1DForOutWhenUnconnected=off
  Psi_dul_dot : Outport  Port=3  VectorParamsAs1DForOutWhenUnconnected=off
  wires:
  Sum4/1 -> Divide1/1
  Theta_dot/1 -> Product/2, Product2/3
  tau_x_1/1 -> Divide3/1
  Sum2/1 -> Psi_dul_dot/1
  Divide6/1 -> Sum1/2
  Sum1/1 -> Theta_dul_dot/1
  tau_z_1/1 -> Divide5/1
  Constant/1 -> Divide3/2, Sum5/1, Sum4/2, Divide/2
  Constant2/1 -> Divide5/2, Divide2/2, Sum4/1, Sum3/2
  Product1/1 -> Sum1/1
  Divide2/1 -> Product2/1
  Psi_dot/1 -> Product1/3, Product/3
  Divide/1 -> Product/1
  Sum5/1 -> Divide2/1
  Sum/1 -> Phi_dul_dot/1
  Divide5/1 -> Sum2/2
  Constant1/1 -> Sum5/2, Divide6/2, Divide1/2, Sum3/1
  Sum3/1 -> Divide/1
  Product/1 -> Sum/1
  Phi_dot/1 -> Product1/2, Product2/2
  Product2/1 -> Sum2/1
  Divide3/1 -> Sum/2
  tau_y_1/1 -> Divide6/1
  Divide1/1 -> Product1/1

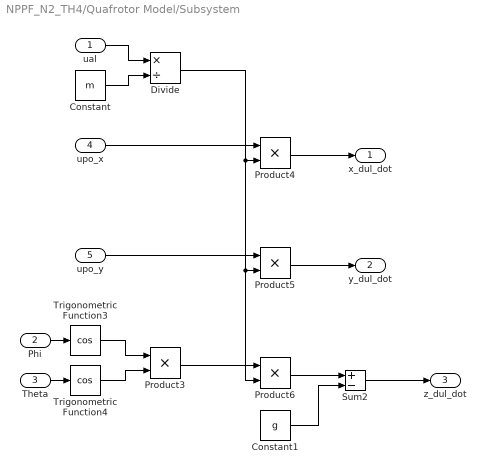
== system NPPF_N2_TH4/Quafrotor Model/Subsystem ==
  ual : Inport
  Phi : Inport  Port=2
  Theta : Inport  Port=3
  upo_x : Inport  Port=4
  upo_y : Inport  Port=5
  Constant : Constant  Value=m
  Constant1 : Constant  Value=g
  Divide : Product  Inputs=*/
  Product{3..6} (4 alike) : Product
  Sum2 : Sum  Inputs=+-
  Trigonometric Function3 : Trigonometry  Operator=cos
  Trigonometric Function4 : Trigonometry  Operator=cos
  x_dul_dot : Outport  VectorParamsAs1DForOutWhenUnconnected=off
  y_dul_dot : Outport  Port=2  VectorParamsAs1DForOutWhenUnconnected=off
  z_dul_dot : Outport  Port=3  VectorParamsAs1DForOutWhenUnconnected=off
  wires:
  Trigonometric Function3/1 -> Product3/1
  Divide/1 -> Product6/2, Product5/2, Product4/2
  Product4/1 -> x_dul_dot/1
  Constant1/1 -> Sum2/2
  Product6/1 -> Sum2/1
  Phi/1 -> Trigonometric Function3/1
  Trigonometric Function4/1 -> Product3/2
  Constant/1 -> Divide/2
  Product3/1 -> Product6/1
  Sum2/1 -> z_dul_dot/1
  Product5/1 -> y_dul_dot/1
  Theta/1 -> Trigonometric Function4/1
  ual/1 -> Divide/1
  upo_x/1 -> Product4/1
  upo_y/1 -> Product5/1

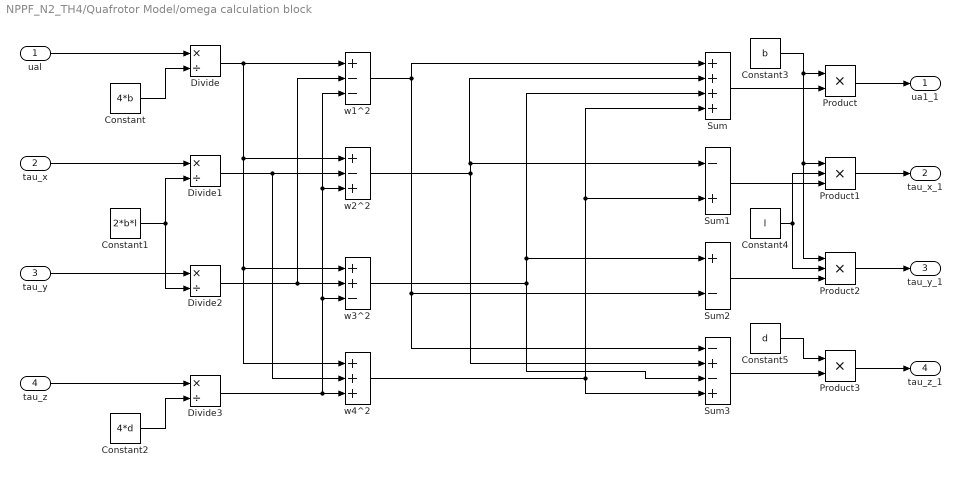
== system NPPF_N2_TH4/Quafrotor Model/omega calculation block ==
  ual : Inport
  tau_x : Inport  Port=2
  tau_y : Inport  Port=3
  tau_z : Inport  Port=4
  Constant : Constant  Value=4*b
  Constant1 : Constant  Value=2*b*l
  Constant2 : Constant  Value=4*d
  Constant3 : Constant  Value=b
  Constant4 : Constant  Value=l
  Constant5 : Constant  Value=d
  Divide{,1..3} (4 alike) : Product  Inputs=*/
  Product : Product
  Product1 : Product  Inputs=3
  Product2 : Product  Inputs=3
  Product3 : Product
  Sum : Sum  Inputs=++++
  Sum1 : Sum  Inputs=-+
  Sum2 : Sum  Inputs=+-
  Sum3 : Sum  Inputs=-+-+
  w1^2 : Sum  Inputs=+--
  w2^2 : Sum  Inputs=+-+
  w3^2 : Sum  Inputs=++-
  w4^2 : Sum  Inputs=+++
  ua1_1 : Outport  VectorParamsAs1DForOutWhenUnconnected=off
  tau_x_1 : Outport  Port=2  VectorParamsAs1DForOutWhenUnconnected=off
  tau_y_1 : Outport  Port=3  VectorParamsAs1DForOutWhenUnconnected=off
  tau_z_1 : Outport  Port=4  VectorParamsAs1DForOutWhenUnconnected=off
  wires:
  w4^2/1 -> Sum3/4, Sum1/2, Sum/4
  Sum3/1 -> Product3/2
  ual/1 -> Divide/1
  Sum2/1 -> Product2/3
  Sum1/1 -> Product1/3
  Constant1/1 -> Divide2/2, Divide1/2
  Divide/1 -> w1^2/1, w2^2/1, w3^2/1, w4^2/1
  Constant5/1 -> Product3/1
  Constant3/1 -> Product2/1, Product1/1, Product/1
  Constant4/1 -> Product1/2, Product2/2
  Product/1 -> ua1_1/1
  w1^2/1 -> Sum/1, Sum2/2, Sum3/1
  w2^2/1 -> Sum1/1, Sum/2, Sum3/2
  tau_x/1 -> Divide1/1
  Product3/1 -> tau_z_1/1
  Divide1/1 -> w2^2/2, w4^2/2
  Divide2/1 -> w3^2/2, w1^2/2
  Divide3/1 -> w4^2/3, w3^2/3, w2^2/3, w1^2/3
  Product2/1 -> tau_y_1/1
  w3^2/1 -> Sum3/3, Sum2/1, Sum/3
  Constant2/1 -> Divide3/2
  Product1/1 -> tau_x_1/1
  tau_y/1 -> Divide2/1
  tau_z/1 -> Divide3/1
  Sum/1 -> Product/2
  Constant/1 -> Divide/2
